simulink model "Flow_Meter_Simulink"  (R2023b)
settings: Solver=FixedStepAuto  StartTime=0.0  StopTime=Stop_Time  RelTol=1e-3
values from neighbouring files (symbols this model uses):
  Sample_Time = (2 * pi) / (Frequency * Samples_Per_Period)    [Flow_Meter_Script.m]
  Stop_Time = input('Enter The Stop Time In Seconds: ')    [Flow_Meter_Script.m]
libraries: commchan3 x1, dspsigops x1
settings Model: Creator=Reaper  LastModifiedBy=Reaper

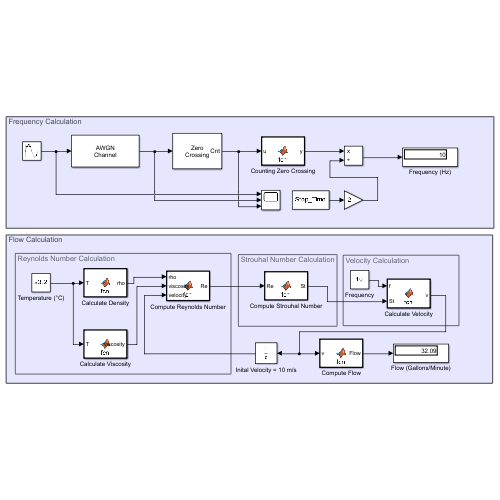
[thumbnail: Simulink's stored preview of the top-level diagram]
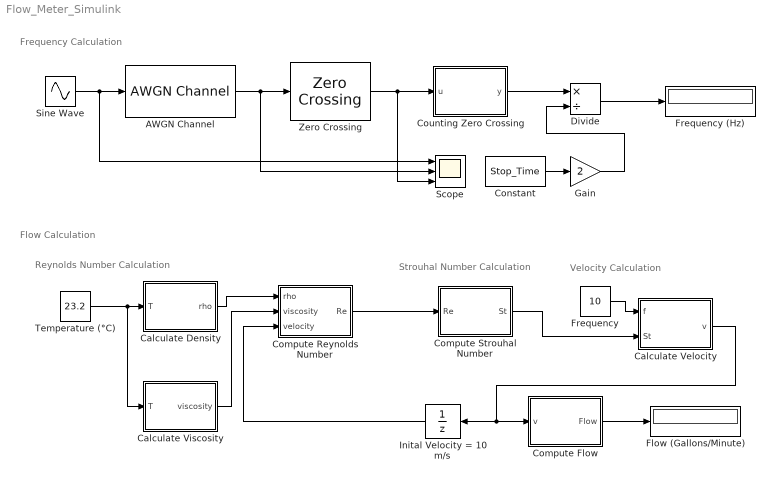
== system Flow_Meter_Simulink ==
  note: Flow Calculation
  note: Velocity Calculation
  note: Frequency Calculation
  note: Reynolds Number Calculation
  note: Strouhal Number Calculation
  AWGN Channel : commchan3/AWGN Channel  LegacyMode=off  NoiseMethod="Signal to noise ratio  (SNR)"  noiseMode="Signal to noise ratio  (SNR)"  EbNo=10  EsNo=10  SNR=20  BitsPerSymbol=1  SignalPower=0.001  SamplesPerSymbol=1  SymbolPeriod=1  VarianceSource=Parameter  Variance=1  RandomStream=Global stream  Seed=67  SimulateUsing=Code generation
  Calculate Density : MATLAB Function  TreatAsAtomicUnit=on
  Calculate Velocity : MATLAB Function  TreatAsAtomicUnit=on
  Calculate Viscosity : MATLAB Function  TreatAsAtomicUnit=on
  Compute Flow : MATLAB Function  TreatAsAtomicUnit=on
  Compute Reynolds Number : MATLAB Function  TreatAsAtomicUnit=on
  Compute Strouhal Number : MATLAB Function  TreatAsAtomicUnit=on
  Constant : Constant  Value=Stop_Time
  Counting Zero Crossing : MATLAB Function  TreatAsAtomicUnit=on
  Divide : Product  Inputs=*/
  Flow (Gallons/Minute) : Display
  Frequency : Constant  Value=10
  Frequency (Hz) : Display
  Gain : Gain  Gain=2
  Inital Velocity = 10 m/s : UnitDelay  InitialCondition=10  SampleTime=-1  HasFrameUpgradeWarning=on
  Scope : Scope  NumInputPorts=3
  Sine Wave : Sin  SineType=Sample based  Frequency=10  Samples=Samples_Per_Period  SampleTime=Sample_Time
  Temperature (°C) : Constant  Value=23.2
  Zero Crossing : dspsigops/Zero Crossing  InputProcessing=Columns as channels (frame based)
  wires:
  Zero Crossing/1 -> Scope/3, Counting Zero Crossing/1(u)
  Counting Zero Crossing/1(y) -> Divide/1
  Divide/1 -> Frequency (Hz)/1
  Constant/1 -> Gain/1
  Gain/1 -> Divide/2
  Sine Wave/1 -> Scope/1, AWGN Channel/1
  AWGN Channel/1 -> Scope/2, Zero Crossing/1
  Calculate Density/1(rho) -> Compute Reynolds Number/1(rho)
  Compute Reynolds Number/1(Re) -> Compute Strouhal Number/1(Re)
  Calculate Velocity/1(v) -> Inital Velocity = 10 m/s/1, Compute Flow/1(v)
  Compute Flow/1(Flow) -> Flow (Gallons/Minute)/1
  Calculate Viscosity/1(viscosity) -> Compute Reynolds Number/2(viscosity)
  Compute Strouhal Number/1(St) -> Calculate Velocity/2(St)
  Temperature (°C)/1 -> Calculate Viscosity/1(T), Calculate Density/1(T)
  Frequency/1 -> Calculate Velocity/1(f)
  Inital Velocity = 10 m/s/1 -> Compute Reynolds Number/3(velocity)

== matlab function Flow_Meter_Simulink/Counting Zero Crossing ==
  data: u input; y output
function y = fcn(u)
    % Persistent variable to keep track of the count
    persistent count;
    
    % Initialize the count variable if it's empty
    if isempty(count)
        count = 0;
    end

    % Increment count if u is greater than 1
    if u == 1
        count = count + 1;
    end
    
    % Output the current count
    y = count;
end

== matlab function Flow_Meter_Simulink/Calculate Viscosity ==
  data: T input; viscosity output
function viscosity = fcn(T)
    T_Kelvin = T + 273.15; % Convert Celsius to Kelvin
    viscosity = 2.4e-5 * 10^(247.8 / (T_Kelvin - 140));
end

== matlab function Flow_Meter_Simulink/Compute Reynolds Number ==
  data: rho input; Re output; viscosity input; velocity input
function Re = fcn(rho, viscosity, velocity)
    %persistent isFirstRun;
    
    %if isempty(isFirstRun)
    %    velocity = 10; % m/s, set the velocity to 10 m/s on the first run
    %    isFirstRun = false;
    %end
    
    PID = 2.900 * 0.0254; % Convert from inches to meters
    Re = (rho * velocity * PID) / viscosity;
end

== matlab function Flow_Meter_Simulink/Compute Strouhal Number ==
  data: Re input; St output
function St = fcn(Re)
    St = 0.2684 - 1.0356 / sqrt(Re);
end

== matlab function Flow_Meter_Simulink/Calculate Velocity ==
  data: f input; v output; St input
function v = fcn(f, St)
    d = 0.5;
    v = f * d / St; % Average fluid velocity in inch per second
end

== matlab function Flow_Meter_Simulink/Compute Flow ==
  data: v input; Flow output
% Compute Flow (in gallons per minute)
function Flow = fcn(v)
    PID = 2.900; % Inner diameter in inches
    v_feet_per_second = v / 12; % Convert velocity from inches/s to feet/s
    Flow = 2.45 * PID^2 * v_feet_per_second;
end

== matlab function Flow_Meter_Simulink/Calculate Density ==
  data: T input; rho output
function rho = fcn(T)
    rho = 1000*(1 - ((T+288.9414)/(508929.2*(T+68.12963)))*(T-3.9863)^2); % in kg/m^3
end
